simulink model "SystemComposerModel"  (R2022b)
settings: Solver=VariableStepAuto  StartTime=0.0  StopTime=10.0  RelTol=1e-3
(part 2 of 3)

== system SystemComposerModel/Crazyflie 2.0/Results ==
  Bus Element In1 : Inport  PortName=Tests
  ResultsAnalysis : Subsystem
      settings: PortSchema="{\"entries\":[{\"content\":{\"headerSize\":26,\"margin\":15,\"minimumSpacing\":25,\"sides\":[{\"content\":{\"connectorIds\":[\"In1\"]},\"type\":\"ConnectorPlacement.EquallySpacedRectSide\",\"uuid\":\"b8d7d09c-e9ae-43de-8d46-f99ec2351e24\"},{\"content\":{\"connectorIds\":[\"Out1\"],\"side\":\"RIGHT\"},\"type\":\"ConnectorPlacement.EquallySpacedRectSide\",\"uuid\":\"4693648e-b0a2-4db8-a983-4bee2f51d894\"},{\"content\":{\"connectorIds\":[],\"side\":\"TOP\"},\"type\":\"ConnectorPlacement.EquallySpacedRectSide\",\"uuid\":\"9f0e5fe3-4fa7-4597-a4df-94b2d5032736\"}]},\"type\":\"ConnectorPlacement.EquallySpacedConnector\",\"uuid\":\"297bf07a-4341-4423-8aed-0af6edbe7857\"}],\"packageUris\":[\"http://schema.mathworks.com/mf0/Connector/R2020b\"],\"version\":\"1.0\"}"
  Bus Element Out1 : Outport  PortName=CodeModifications
  wires:
  Bus Element In1/1 -> ResultsAnalysis/1(Tests)
  ResultsAnalysis/1(CodeModifications) -> Bus Element Out1/1

== system SystemComposerModel/Crazyflie 2.0/STEM ranging ==
  Bus Element Out1 : Outport  PortName=dist_front
  Bus Element Out2 : Outport  Port=2  PortName=dist_rear
  Bus Element Out3 : Outport  Port=3  PortName=dist_right
  Bus Element Out4 : Outport  Port=4  PortName=dist_left

== system SystemComposerModel/Crazyflie 2.0/State Estimator ==
  Bus Element In1 : Inport  PortName=Current state
  Bus Element In2 : Inport  Port=2  PortName=Actuation Signal
  Bus Element Out1 : Outport  PortName=Estimated State

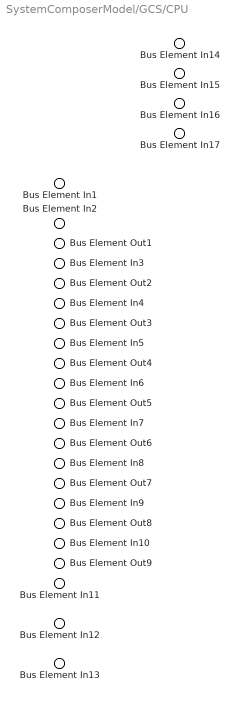
== system SystemComposerModel/GCS/CPU ==
  Bus Element In17 : Inport  PortName=CodeModifications
  Bus Element In14 : Inport  Port=2  PortName=F_x_in
  Bus Element In15 : Inport  Port=3  PortName=F_y_in
  Bus Element In16 : Inport  Port=4  PortName=F_z_in
  Bus Element In1 : Inport  Port=5  PortName=pos_x_in
  Bus Element In2 : Inport  Port=6  PortName=pos_y_in
  Bus Element In3 : Inport  Port=7  PortName=pos_z_in
  Bus Element In4 : Inport  Port=8  PortName=alpha_in
  Bus Element In5 : Inport  Port=9  PortName=beta_in
  Bus Element In6 : Inport  Port=10  PortName=gamma_in
  Bus Element In7 : Inport  Port=11  PortName=vel_x_in
  Bus Element In8 : Inport  Port=12  PortName=vel_y_in
  Bus Element In9 : Inport  Port=13  PortName=vel_z_in
  Bus Element In10 : Inport  Port=14  PortName=Obst_x1_in
  Bus Element In11 : Inport  Port=15  PortName=Obst_y1_in
  Bus Element In12 : Inport  Port=16  PortName=Obst_x2_in
  Bus Element In13 : Inport  Port=17  PortName=Obst_y2_in
  Bus Element Out1 : Outport  PortName=pos_x_out
  Bus Element Out2 : Outport  Port=2  PortName=pos_y_out
  Bus Element Out3 : Outport  Port=3  PortName=pos_z_out
  Bus Element Out4 : Outport  Port=4  PortName=alpha_out
  Bus Element Out5 : Outport  Port=5  PortName=beta_out
  Bus Element Out6 : Outport  Port=6  PortName=gamma_out
  Bus Element Out7 : Outport  Port=7  PortName=vel_x_out
  Bus Element Out8 : Outport  Port=8  PortName=vel_y_out
  Bus Element Out9 : Outport  Port=9  PortName=vel_z_out

== system SystemComposerModel/GCS/ClimConditions ==
  Bus Element In1 : Inport  PortName=Enviroment
  Wind : Subsystem
      settings: PortSchema="{\"entries\":[{\"content\":{\"headerSize\":26,\"margin\":15,\"minimumSpacing\":25,\"sides\":[{\"content\":{\"connectorIds\":[\"In1\"]},\"type\":\"ConnectorPlacement.EquallySpacedRectSide\",\"uuid\":\"b8d7d09c-e9ae-43de-8d46-f99ec2351e24\"},{\"content\":{\"connectorIds\":[\"Out1\",\"Out2\",\"Out3\"],\"side\":\"RIGHT\"},\"type\":\"ConnectorPlacement.EquallySpacedRectSide\",\"uuid\":\"4693648e-b0a2-4db8-a983-4bee2f51d894\"},{\"content\":{\"connectorIds\":[],\"side\":\"TOP\"},\"type\":\"ConnectorPlacement.EquallySpacedRectSide\",\"uuid\":\"9f0e5fe3-4fa7-4597-a4df-94b2d5032736\"}]},\"type\":\"ConnectorPlacement.EquallySpacedConnector\",\"uuid\":\"297bf07a-4341-4423-8aed-0af6edbe7857\"}],\"packageUris\":[\"http://schema.mathworks.com/mf0/Connector/R2020b\"],\"version\":\"1.0\"}"
  Bus Element Out1 : Outport  PortName=F_x_in
  Bus Element Out2 : Outport  Port=2  PortName=F_y_in
  Bus Element Out3 : Outport  Port=3  PortName=F_z_in
  wires:
  Bus Element In1/1 -> Wind/1(Enviroment)
  Wind/1(F_x_in) -> Bus Element Out1/1
  Wind/2(F_y_in) -> Bus Element Out2/1
  Wind/3(F_z_in) -> Bus Element Out3/1

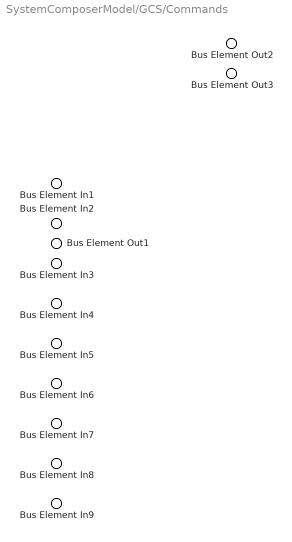
== system SystemComposerModel/GCS/Commands ==
  Bus Element In1 : Inport  PortName=pos_x_out
  Bus Element In2 : Inport  Port=2  PortName=pos_y_out
  Bus Element In3 : Inport  Port=3  PortName=pos_z_out
  Bus Element In4 : Inport  Port=4  PortName=alpha_out
  Bus Element In5 : Inport  Port=5  PortName=beta_out
  Bus Element In6 : Inport  Port=6  PortName=gamma_out
  Bus Element In7 : Inport  Port=7  PortName=vel_x_out
  Bus Element In8 : Inport  Port=8  PortName=vel_y_out
  Bus Element In9 : Inport  Port=9  PortName=vel_z_out
  Bus Element Out2 : Outport  PortName=Telemetry_USB
  Bus Element Out3 : Outport  Port=2  PortName=TelemetryFeedback
  Bus Element Out1 : Outport  Port=3  PortName=GCSCmds

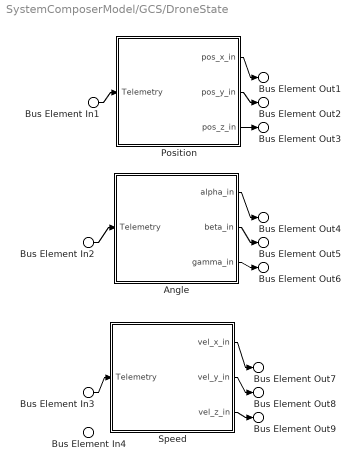
== system SystemComposerModel/GCS/DroneState ==
  Bus Element In1 : Inport  PortName=Telemetry
  Bus Element In2 : Inport  PortName=Telemetry
  Bus Element In3 : Inport  PortName=Telemetry
  Bus Element In4 : Inport  Port=2  PortName=TelemetryFeedback
  Angle : Subsystem
      settings: PortSchema="{\"entries\":[{\"content\":{\"headerSize\":26,\"margin\":15,\"minimumSpacing\":25,\"sides\":[{\"content\":{\"connectorIds\":[\"In1\"]},\"type\":\"ConnectorPlacement.EquallySpacedRectSide\",\"uuid\":\"b8d7d09c-e9ae-43de-8d46-f99ec2351e24\"},{\"content\":{\"connectorIds\":[\"Out1\",\"Out2\",\"Out3\"],\"side\":\"RIGHT\"},\"type\":\"ConnectorPlacement.EquallySpacedRectSide\",\"uuid\":\"4693648e-b0a2-4db8-a983-4bee2f51d894\"},{\"content\":{\"connectorIds\":[],\"side\":\"TOP\"},\"type\":\"ConnectorPlacement.EquallySpacedRectSide\",\"uuid\":\"9f0e5fe3-4fa7-4597-a4df-94b2d5032736\"}]},\"type\":\"ConnectorPlacement.EquallySpacedConnector\",\"uuid\":\"297bf07a-4341-4423-8aed-0af6edbe7857\"}],\"packageUris\":[\"http://schema.mathworks.com/mf0/Connector/R2020b\"],\"version\":\"1.0\"}"
  Position : Subsystem
      settings: PortSchema="{\"entries\":[{\"content\":{\"headerSize\":26,\"margin\":15,\"minimumSpacing\":25,\"sides\":[{\"content\":{\"connectorIds\":[\"In1\"]},\"type\":\"ConnectorPlacement.EquallySpacedRectSide\",\"uuid\":\"b8d7d09c-e9ae-43de-8d46-f99ec2351e24\"},{\"content\":{\"connectorIds\":[\"Out1\",\"Out2\",\"Out3\"],\"side\":\"RIGHT\"},\"type\":\"ConnectorPlacement.EquallySpacedRectSide\",\"uuid\":\"4693648e-b0a2-4db8-a983-4bee2f51d894\"},{\"content\":{\"connectorIds\":[],\"side\":\"TOP\"},\"type\":\"ConnectorPlacement.EquallySpacedRectSide\",\"uuid\":\"9f0e5fe3-4fa7-4597-a4df-94b2d5032736\"}]},\"type\":\"ConnectorPlacement.EquallySpacedConnector\",\"uuid\":\"297bf07a-4341-4423-8aed-0af6edbe7857\"}],\"packageUris\":[\"http://schema.mathworks.com/mf0/Connector/R2020b\"],\"version\":\"1.0\"}"
  Speed : Subsystem
      settings: PortSchema="{\"entries\":[{\"content\":{\"headerSize\":26,\"margin\":15,\"minimumSpacing\":25,\"sides\":[{\"content\":{\"connectorIds\":[\"In1\"]},\"type\":\"ConnectorPlacement.EquallySpacedRectSide\",\"uuid\":\"b8d7d09c-e9ae-43de-8d46-f99ec2351e24\"},{\"content\":{\"connectorIds\":[\"Out1\",\"Out2\",\"Out3\"],\"side\":\"RIGHT\"},\"type\":\"ConnectorPlacement.EquallySpacedRectSide\",\"uuid\":\"4693648e-b0a2-4db8-a983-4bee2f51d894\"},{\"content\":{\"connectorIds\":[],\"side\":\"TOP\"},\"type\":\"ConnectorPlacement.EquallySpacedRectSide\",\"uuid\":\"9f0e5fe3-4fa7-4597-a4df-94b2d5032736\"}]},\"type\":\"ConnectorPlacement.EquallySpacedConnector\",\"uuid\":\"297bf07a-4341-4423-8aed-0af6edbe7857\"}],\"packageUris\":[\"http://schema.mathworks.com/mf0/Connector/R2020b\"],\"version\":\"1.0\"}"
  Bus Element Out1 : Outport  PortName=pos_x_in
  Bus Element Out2 : Outport  Port=2  PortName=pos_y_in
  Bus Element Out3 : Outport  Port=3  PortName=pos_z_in
  Bus Element Out4 : Outport  Port=4  PortName=alpha_in
  Bus Element Out5 : Outport  Port=5  PortName=beta_in
  Bus Element Out6 : Outport  Port=6  PortName=gamma_in
  Bus Element Out7 : Outport  Port=7  PortName=vel_x_in
  Bus Element Out8 : Outport  Port=8  PortName=vel_y_in
  Bus Element Out9 : Outport  Port=9  PortName=vel_z_in
  wires:
  Bus Element In1/1 -> Position/1(Telemetry)
  Bus Element In2/1 -> Angle/1(Telemetry)
  Bus Element In3/1 -> Speed/1(Telemetry)
  Position/1(pos_x_in) -> Bus Element Out1/1
  Position/2(pos_y_in) -> Bus Element Out2/1
  Position/3(pos_z_in) -> Bus Element Out3/1
  Angle/1(alpha_in) -> Bus Element Out4/1
  Angle/2(beta_in) -> Bus Element Out5/1
  Angle/3(gamma_in) -> Bus Element Out6/1
  Speed/1(vel_x_in) -> Bus Element Out7/1
  Speed/2(vel_y_in) -> Bus Element Out8/1
  Speed/3(vel_z_in) -> Bus Element Out9/1

== system SystemComposerModel/GCS/References ==
  Bus Element In1 : Inport  PortName=FPVVideo
  ObstacleDetection : Subsystem
      settings: PortSchema="{\"entries\":[{\"content\":{\"headerSize\":26,\"margin\":15,\"minimumSpacing\":25,\"sides\":[{\"content\":{\"connectorIds\":[\"In1\"]},\"type\":\"ConnectorPlacement.EquallySpacedRectSide\",\"uuid\":\"b8d7d09c-e9ae-43de-8d46-f99ec2351e24\"},{\"content\":{\"connectorIds\":[\"Out1\",\"Out2\",\"Out3\",\"Out4\"],\"side\":\"RIGHT\"},\"type\":\"ConnectorPlacement.EquallySpacedRectSide\",\"uuid\":\"4693648e-b0a2-4db8-a983-4bee2f51d894\"},{\"content\":{\"connectorIds\":[],\"side\":\"TOP\"},\"type\":\"ConnectorPlacement.EquallySpacedRectSide\",\"uuid\":\"9f0e5fe3-4fa7-4597-a4df-94b2d5032736\"}]},\"type\":\"ConnectorPlacement.EquallySpacedConnector\",\"uuid\":\"297bf07a-4341-4423-8aed-0af6edbe7857\"}],\"packageUris\":[\"http://schema.mathworks.com/mf0/Connector/R2020b\"],\"version\":\"1.0\"}"
  Bus Element Out4 : Outport  PortName=Obst_x1_in
  Bus Element Out2 : Outport  Port=2  PortName=Obst_y1_in
  Bus Element Out3 : Outport  Port=3  PortName=Obst_x2_in
  Bus Element Out1 : Outport  Port=4  PortName=Obst_y2_in
  wires:
  Bus Element In1/1 -> ObstacleDetection/1(FPVVideo)
  ObstacleDetection/4(Obst_y2_in) -> Bus Element Out1/1
  ObstacleDetection/3(Obst_y1_in) -> Bus Element Out2/1
  ObstacleDetection/2(Obst_x2_in) -> Bus Element Out3/1
  ObstacleDetection/1(Obst_x1_in) -> Bus Element Out4/1

== system SystemComposerModel/GCS/Results ==
  Bus Element In1 : Inport  PortName=Tests
  ResultsAnalysis : Subsystem
      settings: PortSchema="{\"entries\":[{\"content\":{\"headerSize\":26,\"margin\":15,\"minimumSpacing\":25,\"sides\":[{\"content\":{\"connectorIds\":[\"In1\"]},\"type\":\"ConnectorPlacement.EquallySpacedRectSide\",\"uuid\":\"b8d7d09c-e9ae-43de-8d46-f99ec2351e24\"},{\"content\":{\"connectorIds\":[\"Out1\"],\"side\":\"RIGHT\"},\"type\":\"ConnectorPlacement.EquallySpacedRectSide\",\"uuid\":\"4693648e-b0a2-4db8-a983-4bee2f51d894\"},{\"content\":{\"connectorIds\":[],\"side\":\"TOP\"},\"type\":\"ConnectorPlacement.EquallySpacedRectSide\",\"uuid\":\"9f0e5fe3-4fa7-4597-a4df-94b2d5032736\"}]},\"type\":\"ConnectorPlacement.EquallySpacedConnector\",\"uuid\":\"297bf07a-4341-4423-8aed-0af6edbe7857\"}],\"packageUris\":[\"http://schema.mathworks.com/mf0/Connector/R2020b\"],\"version\":\"1.0\"}"
  Bus Element Out1 : Outport  PortName=CodeModifications
  wires:
  Bus Element In1/1 -> ResultsAnalysis/1(Tests)
  ResultsAnalysis/1(CodeModifications) -> Bus Element Out1/1

== system SystemComposerModel/Competition/Materials/Advertising ==
  Bus Element Out1 : Outport  PortName=Marketing

== system SystemComposerModel/Competition/Materials/Chronometer ==

== system SystemComposerModel/Competition/Materials/Horn ==
  Bus Element Out1 : Outport  PortName=Start

== system SystemComposerModel/Competition/Materials/Insulating tapes ==
  Bus Element Out1 : Outport  PortName=Lines

== system SystemComposerModel/Competition/Materials/Obstacles ==
  Doors : Subsystem  Description=They must be overcome by passing through the middle. The doors will be 1x1 meter square and elevated with the lower base half a meter off the ground.
      settings: PortSchema="{\"entries\":[{\"content\":{\"headerSize\":26,\"margin\":15,\"minimumSpacing\":25,\"sides\":[{\"content\":{\"connectorIds\":[]},\"type\":\"ConnectorPlacement.EquallySpacedRectSide\",\"uuid\":\"9053b2a7-4775-4bcf-9fc6-a069826350a9\"},{\"content\":{\"connectorIds\":[],\"side\":\"RIGHT\"},\"type\":\"ConnectorPlacement.EquallySpacedRectSide\",\"uuid\":\"b0969818-a4d3-4cbe-99b6-1949e99be80f\"},{\"content\":{\"connectorIds\":[],\"side\":\"TOP\"},\"type\":\"ConnectorPlacement.EquallySpacedRectSide\",\"uuid\":\"6c494ee9-6eb7-4ac7-893f-bc2d7701a0da\"}]},\"type\":\"ConnectorPlacement.EquallySpacedConnector\",\"uuid\":\"7a7eacf3-349d-4601-bac9-f57d73c6d0e2\"}],\"packageUris\":[\"http://schema.mathworks.com/mf0/Connector/R2020b\"],\"version\":\"1.0\"}"
  Split Rectangle : Subsystem  Description=They can be red or blue. If they are red, you pass over them and if they are blue, you pass under them. The whole surface of the obstacle will be the same color and each rectangle will be 2x1m.
      settings: PortSchema="{\"entries\":[{\"content\":{\"headerSize\":26,\"margin\":15,\"minimumSpacing\":25,\"sides\":[{\"content\":{\"connectorIds\":[]},\"type\":\"ConnectorPlacement.EquallySpacedRectSide\",\"uuid\":\"9053b2a7-4775-4bcf-9fc6-a069826350a9\"},{\"content\":{\"connectorIds\":[\"Out1\"],\"side\":\"RIGHT\"},\"type\":\"ConnectorPlacement.EquallySpacedRectSide\",\"uuid\":\"b0969818-a4d3-4cbe-99b6-1949e99be80f\"},{\"content\":{\"connectorIds\":[],\"side\":\"TOP\"},\"type\":\"ConnectorPlacement.EquallySpacedRectSide\",\"uuid\":\"6c494ee9-6eb7-4ac7-893f-bc2d7701a0da\"}]},\"type\":\"ConnectorPlacement.EquallySpacedConnector\",\"uuid\":\"7a7eacf3-349d-4601-bac9-f57d73c6d0e2\"}],\"packageUris\":[\"http://schema.mathworks.com/mf0/Connector/R2020b\"],\"version\":\"1.0\"}"
  Sticks : Subsystem  Description=They can be red or blue. If they are red they are passed on the left and if they are blue on the right. The stick will be 1.5 meters long and 4 cm wide. For a correct overcoming of the obstacle, the drone must not move more than 0.5 meters away from the sides and cannot exceed the height of the stick.
      settings: PortSchema="{\"entries\":[{\"content\":{\"headerSize\":26,\"margin\":15,\"minimumSpacing\":25,\"sides\":[{\"content\":{\"connectorIds\":[]},\"type\":\"ConnectorPlacement.EquallySpacedRectSide\",\"uuid\":\"9053b2a7-4775-4bcf-9fc6-a069826350a9\"},{\"content\":{\"connectorIds\":[],\"side\":\"RIGHT\"},\"type\":\"ConnectorPlacement.EquallySpacedRectSide\",\"uuid\":\"b0969818-a4d3-4cbe-99b6-1949e99be80f\"},{\"content\":{\"connectorIds\":[],\"side\":\"TOP\"},\"type\":\"ConnectorPlacement.EquallySpacedRectSide\",\"uuid\":\"6c494ee9-6eb7-4ac7-893f-bc2d7701a0da\"}]},\"type\":\"ConnectorPlacement.EquallySpacedConnector\",\"uuid\":\"7a7eacf3-349d-4601-bac9-f57d73c6d0e2\"}],\"packageUris\":[\"http://schema.mathworks.com/mf0/Connector/R2020b\"],\"version\":\"1.0\"}"
  Bus Element Out1 : Outport  PortName=obs
  wires:
  Split Rectangle/1(OutBus) -> Bus Element Out1/1

== system SystemComposerModel/Competition/Materials/Projector ==
  Bus Element Out1 : Outport  PortName=Proyection

== system SystemComposerModel/Competition/Organization/Before the competition ==
  Marketing : Subsystem  Description=Tasks related to the marketing of the event. Must be started at most 2 weeks before the event.
      settings: PortSchema="{\"entries\":[{\"content\":{\"headerSize\":26,\"margin\":15,\"minimumSpacing\":25,\"sides\":[{\"content\":{\"connectorIds\":[]},\"type\":\"ConnectorPlacement.EquallySpacedRectSide\",\"uuid\":\"d34c32ef-3d27-469b-8a35-abebe5333993\"},{\"content\":{\"connectorIds\":[],\"side\":\"RIGHT\"},\"type\":\"ConnectorPlacement.EquallySpacedRectSide\",\"uuid\":\"0a2917af-f234-4cdf-997c-680a118988b7\"},{\"content\":{\"connectorIds\":[],\"side\":\"TOP\"},\"type\":\"ConnectorPlacement.EquallySpacedRectSide\",\"uuid\":\"dcac7d54-9fff-4582-ba14-08bcbac36cd8\"}]},\"type\":\"ConnectorPlacement.EquallySpacedConnector\",\"uuid\":\"84591ee6-ffcc-49ff-97f7-997353b331d9\"}],\"packageUris\":[\"http://schema.mathworks.com/mf0/Connector/R2020b\"],\"version\":\"1.0\"}"
  Space reservation : Subsystem  Description=Must be done 2 month before the start of the event.
      settings: PortSchema="{\"entries\":[{\"content\":{\"headerSize\":26,\"margin\":15,\"minimumSpacing\":25,\"sides\":[{\"content\":{\"connectorIds\":[]},\"type\":\"ConnectorPlacement.EquallySpacedRectSide\",\"uuid\":\"d34c32ef-3d27-469b-8a35-abebe5333993\"},{\"content\":{\"connectorIds\":[],\"side\":\"RIGHT\"},\"type\":\"ConnectorPlacement.EquallySpacedRectSide\",\"uuid\":\"0a2917af-f234-4cdf-997c-680a118988b7\"},{\"content\":{\"connectorIds\":[],\"side\":\"TOP\"},\"type\":\"ConnectorPlacement.EquallySpacedRectSide\",\"uuid\":\"dcac7d54-9fff-4582-ba14-08bcbac36cd8\"}]},\"type\":\"ConnectorPlacement.EquallySpacedConnector\",\"uuid\":\"84591ee6-ffcc-49ff-97f7-997353b331d9\"}],\"packageUris\":[\"http://schema.mathworks.com/mf0/Connector/R2020b\"],\"version\":\"1.0\"}"

== system SystemComposerModel/Competition/Organization/During the competition ==
  Date : Subsystem  Description=To be defined. It will be at the end of the course.
      settings: PortSchema="{\"entries\":[{\"content\":{\"headerSize\":26,\"margin\":15,\"minimumSpacing\":25,\"sides\":[{\"content\":{\"connectorIds\":[]},\"type\":\"ConnectorPlacement.EquallySpacedRectSide\",\"uuid\":\"d34c32ef-3d27-469b-8a35-abebe5333993\"},{\"content\":{\"connectorIds\":[],\"side\":\"RIGHT\"},\"type\":\"ConnectorPlacement.EquallySpacedRectSide\",\"uuid\":\"0a2917af-f234-4cdf-997c-680a118988b7\"},{\"content\":{\"connectorIds\":[],\"side\":\"TOP\"},\"type\":\"ConnectorPlacement.EquallySpacedRectSide\",\"uuid\":\"dcac7d54-9fff-4582-ba14-08bcbac36cd8\"}]},\"type\":\"ConnectorPlacement.EquallySpacedConnector\",\"uuid\":\"84591ee6-ffcc-49ff-97f7-997353b331d9\"}],\"packageUris\":[\"http://schema.mathworks.com/mf0/Connector/R2020b\"],\"version\":\"1.0\"}"
  Place : Subsystem  Description=Place of the event. It will be the sports centre of ETSII.
      settings: PortSchema="{\"entries\":[{\"content\":{\"headerSize\":26,\"margin\":15,\"minimumSpacing\":25,\"sides\":[{\"content\":{\"connectorIds\":[]},\"type\":\"ConnectorPlacement.EquallySpacedRectSide\",\"uuid\":\"d34c32ef-3d27-469b-8a35-abebe5333993\"},{\"content\":{\"connectorIds\":[],\"side\":\"RIGHT\"},\"type\":\"ConnectorPlacement.EquallySpacedRectSide\",\"uuid\":\"0a2917af-f234-4cdf-997c-680a118988b7\"},{\"content\":{\"connectorIds\":[],\"side\":\"TOP\"},\"type\":\"ConnectorPlacement.EquallySpacedRectSide\",\"uuid\":\"dcac7d54-9fff-4582-ba14-08bcbac36cd8\"}]},\"type\":\"ConnectorPlacement.EquallySpacedConnector\",\"uuid\":\"84591ee6-ffcc-49ff-97f7-997353b331d9\"}],\"packageUris\":[\"http://schema.mathworks.com/mf0/Connector/R2020b\"],\"version\":\"1.0\"}"
  Schedule : Subsystem  Description=The schedule for the different activities of the event. To be defined.
      settings: PortSchema="{\"entries\":[{\"content\":{\"headerSize\":26,\"margin\":15,\"minimumSpacing\":25,\"sides\":[{\"content\":{\"connectorIds\":[]},\"type\":\"ConnectorPlacement.EquallySpacedRectSide\",\"uuid\":\"d34c32ef-3d27-469b-8a35-abebe5333993\"},{\"content\":{\"connectorIds\":[],\"side\":\"RIGHT\"},\"type\":\"ConnectorPlacement.EquallySpacedRectSide\",\"uuid\":\"0a2917af-f234-4cdf-997c-680a118988b7\"},{\"content\":{\"connectorIds\":[],\"side\":\"TOP\"},\"type\":\"ConnectorPlacement.EquallySpacedRectSide\",\"uuid\":\"dcac7d54-9fff-4582-ba14-08bcbac36cd8\"}]},\"type\":\"ConnectorPlacement.EquallySpacedConnector\",\"uuid\":\"84591ee6-ffcc-49ff-97f7-997353b331d9\"}],\"packageUris\":[\"http://schema.mathworks.com/mf0/Connector/R2020b\"],\"version\":\"1.0\"}"

== system SystemComposerModel/Competition/People/Audience ==

== system SystemComposerModel/Competition/People/Observers ==

== system SystemComposerModel/Competition/People/Participants ==

== system SystemComposerModel/Competition/Trials/Prueba 1: Speed ==
  Bus Element In1 : Inport  PortName=Start
  Rules : Subsystem  Description=|
      | The two drones will compete simultaneously, at a distance of at least 5 meters from each other and from the enclosure boundaries.
      | No AI deck or camera is required in this test. 
      | Take-off when the start signal is given, which will consist of a horn sound.
      | Collision between drones means expulsion from the test of the drone that has deviated from the straight line (can be both).
      | The drones must be able to brake so as not to collide with the end of the pavilion. The contestants will calculate the time of power-on of the drone taking into account its maximum speed and the length of the pavilion.
      | Landing after braking.
      | The drone will be disqualified from the test if it takes off before the horn.
      | A time keeper from each team will be stationed at the end of the straight with a stopwatch to mark the finish time. If there is a difference of more than 0.3s between stopwatches the race will be repeated (to avoid cheating).
      settings: PortSchema="{\"entries\":[{\"content\":{\"headerSize\":26,\"margin\":15,\"minimumSpacing\":25,\"sides\":[{\"content\":{\"connectorIds\":[]},\"type\":\"ConnectorPlacement.EquallySpacedRectSide\",\"uuid\":\"9053b2a7-4775-4bcf-9fc6-a069826350a9\"},{\"content\":{\"connectorIds\":[],\"side\":\"RIGHT\"},\"type\":\"ConnectorPlacement.EquallySpacedRectSide\",\"uuid\":\"b0969818-a4d3-4cbe-99b6-1949e99be80f\"},{\"content\":{\"connectorIds\":[],\"side\":\"TOP\"},\"type\":\"ConnectorPlacement.EquallySpacedRectSide\",\"uuid\":\"6c494ee9-6eb7-4ac7-893f-bc2d7701a0da\"}]},\"type\":\"ConnectorPlacement.EquallySpacedConnector\",\"uuid\":\"7a7eacf3-349d-4601-bac9-f57d73c6d0e2\"}],\"packageUris\":[\"http://schema.mathworks.com/mf0/Connector/R2020b\"],\"version\":\"1.0\"}"
  Scoring : Subsystem  Description=|
      | The correct take-off/landing will be analyzed.
      | In this test what determines the score is the time that separates the landing from the take-off, having traveled the length of the pavilion between both maneuvers.
      | The first drone to land after crossing the finish line is considered the winner.
      | A score of 20 points will be awarded to the winning drone and 10 to the losing drone, regardless of the difference that may exist in the times of one and the other. In case of a tie, 15 points will be given to each.
      settings: PortSchema="{\"entries\":[{\"content\":{\"headerSize\":26,\"margin\":15,\"minimumSpacing\":25,\"sides\":[{\"content\":{\"connectorIds\":[]},\"type\":\"ConnectorPlacement.EquallySpacedRectSide\",\"uuid\":\"9053b2a7-4775-4bcf-9fc6-a069826350a9\"},{\"content\":{\"connectorIds\":[],\"side\":\"RIGHT\"},\"type\":\"ConnectorPlacement.EquallySpacedRectSide\",\"uuid\":\"b0969818-a4d3-4cbe-99b6-1949e99be80f\"},{\"content\":{\"connectorIds\":[],\"side\":\"TOP\"},\"type\":\"ConnectorPlacement.EquallySpacedRectSide\",\"uuid\":\"6c494ee9-6eb7-4ac7-893f-bc2d7701a0da\"}]},\"type\":\"ConnectorPlacement.EquallySpacedConnector\",\"uuid\":\"7a7eacf3-349d-4601-bac9-f57d73c6d0e2\"}],\"packageUris\":[\"http://schema.mathworks.com/mf0/Connector/R2020b\"],\"version\":\"1.0\"}"

== system SystemComposerModel/Competition/Trials/Prueba 2: Diana ==
  Bus Element In1 : Inport  PortName=Proyection
  Rules : Subsystem  Description=|
      | Drone takes off when it sees green light on the projector, the screen will turn green for 5 seconds, and the drone will be waiting for the circles.
      | Drone lands when it sees red light on the screen, the screen will turn red for 5 seconds.
      | During 1 minute, one by one black filled circles of 10 cm diameter will be projected consecutively on a wall in an area of 3x2 meters. Each circle will be visible between 4 and 8 seconds, and its position will not be known beforehand but will be the same for both teams.
      | The projector will be 2 meters away from the wall and on the floor, at an angle that makes the projection possible and leaving the drone a maneuvering area such that it does not get in front of the projector.
      | The drone will be disqualified from the event if it covers the projector.
      | Two observers, one from each team, will count the hits. The laser must stay at least an appreciable time inside the circle to count as a hit, it is not enough to pass over it as it may be chance and not the result of the drone's computation.
      settings: PortSchema="{\"entries\":[{\"content\":{\"headerSize\":26,\"margin\":15,\"minimumSpacing\":25,\"sides\":[{\"content\":{\"connectorIds\":[]},\"type\":\"ConnectorPlacement.EquallySpacedRectSide\",\"uuid\":\"9053b2a7-4775-4bcf-9fc6-a069826350a9\"},{\"content\":{\"connectorIds\":[],\"side\":\"RIGHT\"},\"type\":\"ConnectorPlacement.EquallySpacedRectSide\",\"uuid\":\"b0969818-a4d3-4cbe-99b6-1949e99be80f\"},{\"content\":{\"connectorIds\":[],\"side\":\"TOP\"},\"type\":\"ConnectorPlacement.EquallySpacedRectSide\",\"uuid\":\"6c494ee9-6eb7-4ac7-893f-bc2d7701a0da\"}]},\"type\":\"ConnectorPlacement.EquallySpacedConnector\",\"uuid\":\"7a7eacf3-349d-4601-bac9-f57d73c6d0e2\"}],\"packageUris\":[\"http://schema.mathworks.com/mf0/Connector/R2020b\"],\"version\":\"1.0\"}"
  Scoring : Subsystem  Description=|
      | Highest number of hits while aiming at the target.
      | Disqualification in case of obstructing the projection of the targets.
      | The maximum score of the test is 20 points.
      | In this test all the circles will have the same score, so that 20/x points will be added (x being the number of total circles that will appear) each time the laser is placed on a circle at least the stipulated time. 
      | Even if a drone gets the score for a certain circle, the other drone will also be able to get the score for the same circle even if it has put its laser on it later.
      settings: PortSchema="{\"entries\":[{\"content\":{\"headerSize\":26,\"margin\":15,\"minimumSpacing\":25,\"sides\":[{\"content\":{\"connectorIds\":[]},\"type\":\"ConnectorPlacement.EquallySpacedRectSide\",\"uuid\":\"9053b2a7-4775-4bcf-9fc6-a069826350a9\"},{\"content\":{\"connectorIds\":[],\"side\":\"RIGHT\"},\"type\":\"ConnectorPlacement.EquallySpacedRectSide\",\"uuid\":\"b0969818-a4d3-4cbe-99b6-1949e99be80f\"},{\"content\":{\"connectorIds\":[],\"side\":\"TOP\"},\"type\":\"ConnectorPlacement.EquallySpacedRectSide\",\"uuid\":\"6c494ee9-6eb7-4ac7-893f-bc2d7701a0da\"}]},\"type\":\"ConnectorPlacement.EquallySpacedConnector\",\"uuid\":\"7a7eacf3-349d-4601-bac9-f57d73c6d0e2\"}],\"packageUris\":[\"http://schema.mathworks.com/mf0/Connector/R2020b\"],\"version\":\"1.0\"}"

== system SystemComposerModel/Competition/Trials/Prueba 3: Line following ==
  Bus Element In2 : Inport  PortName=Líneas
  Bus Element In1 : Inport  Port=2  PortName=Start
  Rules : Subsystem  Description=|
      | The drone takes off when the start signal is given, which will consist of a horn sound.
      | The drone must follow a continuous black line 38mm wide from start to finish. 
      | The drone must pass through checkpoints (to be defined when the circuit is created) to avoid cheating shortcuts.
      | The circuit will not be known by the teams in advance, it will be random.
      | There will be two types of possible bifurcations:
      | Thinner black line, representing a distraction to avoid, 10mm wide.
      | Red line 20mm wide, which represents the optimal route, thus giving a higher score.
      | The lines shall be sufficiently far apart so as not to confuse the camera.
      | Lines may not cross each other.
      | Landing when a blue tape mark is detected.
      settings: PortSchema="{\"entries\":[{\"content\":{\"headerSize\":26,\"margin\":15,\"minimumSpacing\":25,\"sides\":[{\"content\":{\"connectorIds\":[]},\"type\":\"ConnectorPlacement.EquallySpacedRectSide\",\"uuid\":\"9053b2a7-4775-4bcf-9fc6-a069826350a9\"},{\"content\":{\"connectorIds\":[],\"side\":\"RIGHT\"},\"type\":\"ConnectorPlacement.EquallySpacedRectSide\",\"uuid\":\"b0969818-a4d3-4cbe-99b6-1949e99be80f\"},{\"content\":{\"connectorIds\":[],\"side\":\"TOP\"},\"type\":\"ConnectorPlacement.EquallySpacedRectSide\",\"uuid\":\"6c494ee9-6eb7-4ac7-893f-bc2d7701a0da\"}]},\"type\":\"ConnectorPlacement.EquallySpacedConnector\",\"uuid\":\"7a7eacf3-349d-4601-bac9-f57d73c6d0e2\"}],\"packageUris\":[\"http://schema.mathworks.com/mf0/Connector/R2020b\"],\"version\":\"1.0\"}"
  Scoring : Subsystem  Description=|
      | In this test, drones are awarded points for following a line. When the drone leaves the line it will be given the score of the last control point; from that moment on it is not possible to continue scoring even if the drone recovers the trajectory of the line.
      | To run the complete circuit through the thickest lines possible will result in obtaining the maximum possible score in the test, which will be 18 points.
      | The thickness of the line indicates the score that gives a given section to the next control point. To obtain the score, the area of the lines traversed (thickness * length) is calculated, multiplied by 18 and divided by the area of the lines of the highest scoring path.
      | If you land correctly, you will get 2 extra points, so you can get up to 20 points in this test.
      settings: PortSchema="{\"entries\":[{\"content\":{\"headerSize\":26,\"margin\":15,\"minimumSpacing\":25,\"sides\":[{\"content\":{\"connectorIds\":[]},\"type\":\"ConnectorPlacement.EquallySpacedRectSide\",\"uuid\":\"9053b2a7-4775-4bcf-9fc6-a069826350a9\"},{\"content\":{\"connectorIds\":[],\"side\":\"RIGHT\"},\"type\":\"ConnectorPlacement.EquallySpacedRectSide\",\"uuid\":\"b0969818-a4d3-4cbe-99b6-1949e99be80f\"},{\"content\":{\"connectorIds\":[],\"side\":\"TOP\"},\"type\":\"ConnectorPlacement.EquallySpacedRectSide\",\"uuid\":\"6c494ee9-6eb7-4ac7-893f-bc2d7701a0da\"}]},\"type\":\"ConnectorPlacement.EquallySpacedConnector\",\"uuid\":\"7a7eacf3-349d-4601-bac9-f57d73c6d0e2\"}],\"packageUris\":[\"http://schema.mathworks.com/mf0/Connector/R2020b\"],\"version\":\"1.0\"}"

== system SystemComposerModel/Competition/Trials/Prueba 4: Predefined Obstacles ==
  Bus Element In2 : Inport  PortName=Start
  Bus Element In1 : Inport  Port=2  PortName=Obstacles
  Rules : Subsystem  Description=|
      | Take-off when the departure signal is given, which will consist of a horn sound.
      | Landing when the bidi code of the last obstacle is detected.
      | Provided there is no obstacle present, the drone should be kept at a height of approximately 1m.
      | If an obstacle is omitted it will be considered erroneous.
      | The route must be completed in less than 4 minutes.
      settings: PortSchema="{\"entries\":[{\"content\":{\"headerSize\":26,\"margin\":15,\"minimumSpacing\":25,\"sides\":[{\"content\":{\"connectorIds\":[]},\"type\":\"ConnectorPlacement.EquallySpacedRectSide\",\"uuid\":\"9053b2a7-4775-4bcf-9fc6-a069826350a9\"},{\"content\":{\"connectorIds\":[],\"side\":\"RIGHT\"},\"type\":\"ConnectorPlacement.EquallySpacedRectSide\",\"uuid\":\"b0969818-a4d3-4cbe-99b6-1949e99be80f\"},{\"content\":{\"connectorIds\":[],\"side\":\"TOP\"},\"type\":\"ConnectorPlacement.EquallySpacedRectSide\",\"uuid\":\"6c494ee9-6eb7-4ac7-893f-bc2d7701a0da\"}]},\"type\":\"ConnectorPlacement.EquallySpacedConnector\",\"uuid\":\"7a7eacf3-349d-4601-bac9-f57d73c6d0e2\"}],\"packageUris\":[\"http://schema.mathworks.com/mf0/Connector/R2020b\"],\"version\":\"1.0\"}"
  Scoring : Subsystem  Description=|
      | Test with obstacles (predefined and random): the score at the start of the race is zero points. 
      | Each obstacle passed adds one point. 
      | If the time between two obstacles of one team is at least 0.25 seconds shorter than the time between the same obstacles of the other team, the team with the shorter time will score an additional point (to avoid very close results, where the reaction time of the observers is very important). 
      | To measure the times, two observers will be designated (one of them will be an observer). Two observers (one from each team) will be designated for each obstacle. Their function will be to time the moment when the drone crosses the obstacle. At the start of the race, all observers will start a stopwatch on their mobile devices and stop it when the drone passes the obstacle. If the difference between the times of the two observers is less than 0.2 seconds, the average of the two times will be taken. If this is not the case, this time will not be taken into account for both teams, but the time between two non-consecutive obstacles (with the invalidated one in between) will be taken into account.
      settings: PortSchema="{\"entries\":[{\"content\":{\"headerSize\":26,\"margin\":15,\"minimumSpacing\":25,\"sides\":[{\"content\":{\"connectorIds\":[]},\"type\":\"ConnectorPlacement.EquallySpacedRectSide\",\"uuid\":\"9053b2a7-4775-4bcf-9fc6-a069826350a9\"},{\"content\":{\"connectorIds\":[],\"side\":\"RIGHT\"},\"type\":\"ConnectorPlacement.EquallySpacedRectSide\",\"uuid\":\"b0969818-a4d3-4cbe-99b6-1949e99be80f\"},{\"content\":{\"connectorIds\":[],\"side\":\"TOP\"},\"type\":\"ConnectorPlacement.EquallySpacedRectSide\",\"uuid\":\"6c494ee9-6eb7-4ac7-893f-bc2d7701a0da\"}]},\"type\":\"ConnectorPlacement.EquallySpacedConnector\",\"uuid\":\"7a7eacf3-349d-4601-bac9-f57d73c6d0e2\"}],\"packageUris\":[\"http://schema.mathworks.com/mf0/Connector/R2020b\"],\"version\":\"1.0\"}"
  Trial Obstacles : Subsystem
      settings: PortSchema="{\"entries\":[{\"content\":{\"headerSize\":26,\"margin\":15,\"minimumSpacing\":25,\"sides\":[{\"content\":{\"connectorIds\":[\"In1\"]},\"type\":\"ConnectorPlacement.EquallySpacedRectSide\",\"uuid\":\"9053b2a7-4775-4bcf-9fc6-a069826350a9\"},{\"content\":{\"connectorIds\":[],\"side\":\"RIGHT\"},\"type\":\"ConnectorPlacement.EquallySpacedRectSide\",\"uuid\":\"b0969818-a4d3-4cbe-99b6-1949e99be80f\"},{\"content\":{\"connectorIds\":[],\"side\":\"TOP\"},\"type\":\"ConnectorPlacement.EquallySpacedRectSide\",\"uuid\":\"6c494ee9-6eb7-4ac7-893f-bc2d7701a0da\"}]},\"type\":\"ConnectorPlacement.EquallySpacedConnector\",\"uuid\":\"7a7eacf3-349d-4601-bac9-f57d73c6d0e2\"}],\"packageUris\":[\"http://schema.mathworks.com/mf0/Connector/R2020b\"],\"version\":\"1.0\"}"
  wires:
  Bus Element In1/1 -> Trial Obstacles/1(Obstacles)

== system SystemComposerModel/Competition/Trials/Prueba 5: Random obstacles ==
  Bus Element In2 : Inport  PortName=Start
  Bus Element In1 : Inport  Port=2  PortName=Obstacles
  Rules : Subsystem  Description=|
      | The obstacles will be random.
      | Take-off when the start signal is given, which will consist of a horn sound.
      | Landing when the bidi code of the last obstacle is detected.
      | Test with obstacles (predefined and random): the score at the start of the race is zero points. 
      | Each obstacle passed adds one point. 
      | If the time between two obstacles of one team is at least 0.25 seconds less than the time between the same obstacles of the other team, the team with the shorter time will score an additional point (to avoid very close results, where the reaction time of the observers is very important). 
      | To measure the times, two observers will be designated (one of them will be an observer). Two observers (one from each team) will be designated for each obstacle. Their function will be to time the moment when the drone crosses the obstacle. At the start of the race, all observers will start a stopwatch on their mobile devices and stop it when the drone passes the obstacle. If the difference between the times of the two observers is less than 0.2 seconds, the average of the two times will be taken. If this is not the case, this time will not be taken into account for both teams, but the time between two non-consecutive obstacles (with the invalidated one in between) will be taken into account.
      settings: PortSchema="{\"entries\":[{\"content\":{\"headerSize\":26,\"margin\":15,\"minimumSpacing\":25,\"sides\":[{\"content\":{\"connectorIds\":[]},\"type\":\"ConnectorPlacement.EquallySpacedRectSide\",\"uuid\":\"9053b2a7-4775-4bcf-9fc6-a069826350a9\"},{\"content\":{\"connectorIds\":[],\"side\":\"RIGHT\"},\"type\":\"ConnectorPlacement.EquallySpacedRectSide\",\"uuid\":\"b0969818-a4d3-4cbe-99b6-1949e99be80f\"},{\"content\":{\"connectorIds\":[],\"side\":\"TOP\"},\"type\":\"ConnectorPlacement.EquallySpacedRectSide\",\"uuid\":\"6c494ee9-6eb7-4ac7-893f-bc2d7701a0da\"}]},\"type\":\"ConnectorPlacement.EquallySpacedConnector\",\"uuid\":\"7a7eacf3-349d-4601-bac9-f57d73c6d0e2\"}],\"packageUris\":[\"http://schema.mathworks.com/mf0/Connector/R2020b\"],\"version\":\"1.0\"}"
  Scoring : Subsystem  Description=|
      | Test with obstacles (predefined and random): the score at the start of the race is zero points. 
      | Each obstacle passed adds one point. 
      | If the time between two obstacles of one team is at least 0.25 seconds shorter than the time between the same obstacles of the other team, the team with the shorter time will score an additional point (to avoid very close results, where the reaction time of the observers is very important). 
      | To measure the times, two observers will be designated (one of them will be an observer). Two observers (one from each team) will be designated for each obstacle. Their function will be to time the moment when the drone crosses the obstacle. At the start of the race, all observers will start a stopwatch on their mobile devices and stop it when the drone passes the obstacle. If the difference between the times of the two observers is less than 0.2 seconds, the average of the two times will be taken. If this is not the case, this time will not be taken into account for both teams, but the time between two non-consecutive obstacles (with the invalidated one in between) will be taken into account.
      settings: PortSchema="{\"entries\":[{\"content\":{\"headerSize\":26,\"margin\":15,\"minimumSpacing\":25,\"sides\":[{\"content\":{\"connectorIds\":[]},\"type\":\"ConnectorPlacement.EquallySpacedRectSide\",\"uuid\":\"9053b2a7-4775-4bcf-9fc6-a069826350a9\"},{\"content\":{\"connectorIds\":[],\"side\":\"RIGHT\"},\"type\":\"ConnectorPlacement.EquallySpacedRectSide\",\"uuid\":\"b0969818-a4d3-4cbe-99b6-1949e99be80f\"},{\"content\":{\"connectorIds\":[],\"side\":\"TOP\"},\"type\":\"ConnectorPlacement.EquallySpacedRectSide\",\"uuid\":\"6c494ee9-6eb7-4ac7-893f-bc2d7701a0da\"}]},\"type\":\"ConnectorPlacement.EquallySpacedConnector\",\"uuid\":\"7a7eacf3-349d-4601-bac9-f57d73c6d0e2\"}],\"packageUris\":[\"http://schema.mathworks.com/mf0/Connector/R2020b\"],\"version\":\"1.0\"}"
  Trial Obstacles1 : Subsystem
      settings: PortSchema="{\"entries\":[{\"content\":{\"headerSize\":26,\"margin\":15,\"minimumSpacing\":25,\"sides\":[{\"content\":{\"connectorIds\":[\"In1\"]},\"type\":\"ConnectorPlacement.EquallySpacedRectSide\",\"uuid\":\"9053b2a7-4775-4bcf-9fc6-a069826350a9\"},{\"content\":{\"connectorIds\":[],\"side\":\"RIGHT\"},\"type\":\"ConnectorPlacement.EquallySpacedRectSide\",\"uuid\":\"b0969818-a4d3-4cbe-99b6-1949e99be80f\"},{\"content\":{\"connectorIds\":[],\"side\":\"TOP\"},\"type\":\"ConnectorPlacement.EquallySpacedRectSide\",\"uuid\":\"6c494ee9-6eb7-4ac7-893f-bc2d7701a0da\"}]},\"type\":\"ConnectorPlacement.EquallySpacedConnector\",\"uuid\":\"7a7eacf3-349d-4601-bac9-f57d73c6d0e2\"}],\"packageUris\":[\"http://schema.mathworks.com/mf0/Connector/R2020b\"],\"version\":\"1.0\"}"

== system SystemComposerModel/Competition/Trials/Prueba 6: Freestyle ==
  Bus Element In1 : Inport  PortName=Start
  Rules : Subsystem  Description=Both teams will perform it separately.
      settings: PortSchema="{\"entries\":[{\"content\":{\"headerSize\":26,\"margin\":15,\"minimumSpacing\":25,\"sides\":[{\"content\":{\"connectorIds\":[]},\"type\":\"ConnectorPlacement.EquallySpacedRectSide\",\"uuid\":\"9053b2a7-4775-4bcf-9fc6-a069826350a9\"},{\"content\":{\"connectorIds\":[],\"side\":\"RIGHT\"},\"type\":\"ConnectorPlacement.EquallySpacedRectSide\",\"uuid\":\"b0969818-a4d3-4cbe-99b6-1949e99be80f\"},{\"content\":{\"connectorIds\":[],\"side\":\"TOP\"},\"type\":\"ConnectorPlacement.EquallySpacedRectSide\",\"uuid\":\"6c494ee9-6eb7-4ac7-893f-bc2d7701a0da\"}]},\"type\":\"ConnectorPlacement.EquallySpacedConnector\",\"uuid\":\"7a7eacf3-349d-4601-bac9-f57d73c6d0e2\"}],\"packageUris\":[\"http://schema.mathworks.com/mf0/Connector/R2020b\"],\"version\":\"1.0\"}"

== system SystemComposerModel/Crazyflie 2.0/ClimConditions/Wind ==
  Bus Element In1 : Inport  PortName=Enviroment
  Bus Element Out1 : Outport  PortName=F_x_in
  Bus Element Out2 : Outport  Port=2  PortName=F_y_in
  Bus Element Out3 : Outport  Port=3  PortName=F_z_in

== system SystemComposerModel/Crazyflie 2.0/Results/ResultsAnalysis ==
  Bus Element In1 : Inport  PortName=Tests
  Bus Element Out1 : Outport  PortName=CodeModifications

== system SystemComposerModel/GCS/ClimConditions/Wind ==
  Bus Element In1 : Inport  PortName=Enviroment
  Bus Element Out1 : Outport  PortName=F_x_in
  Bus Element Out2 : Outport  Port=2  PortName=F_y_in
  Bus Element Out3 : Outport  Port=3  PortName=F_z_in

== system SystemComposerModel/GCS/DroneState/Angle ==
  Bus Element In1 : Inport  PortName=Telemetry
  Bus Element Out1 : Outport  PortName=alpha_in
  Bus Element Out2 : Outport  Port=2  PortName=beta_in
  Bus Element Out3 : Outport  Port=3  PortName=gamma_in

== system SystemComposerModel/GCS/DroneState/Position ==
  Bus Element In1 : Inport  PortName=Telemetry
  Bus Element Out1 : Outport  PortName=pos_x_in
  Bus Element Out2 : Outport  Port=2  PortName=pos_y_in
  Bus Element Out3 : Outport  Port=3  PortName=pos_z_in

== system SystemComposerModel/GCS/DroneState/Speed ==
  Bus Element In1 : Inport  PortName=Telemetry
  Bus Element Out1 : Outport  PortName=vel_x_in
  Bus Element Out2 : Outport  Port=2  PortName=vel_y_in
  Bus Element Out3 : Outport  Port=3  PortName=vel_z_in

== system SystemComposerModel/GCS/References/ObstacleDetection ==
  Bus Element In1 : Inport  PortName=FPVVideo
  Bus Element Out1 : Outport  PortName=Obst_x1_in
  Bus Element Out2 : Outport  Port=2  PortName=Obst_x2_in
  Bus Element Out3 : Outport  Port=3  PortName=Obst_y1_in
  Bus Element Out4 : Outport  Port=4  PortName=Obst_y2_in

== system SystemComposerModel/GCS/Results/ResultsAnalysis ==
  Bus Element In1 : Inport  PortName=Tests
  Bus Element Out1 : Outport  PortName=CodeModifications

== system SystemComposerModel/Competition/Materials/Obstacles/Doors ==

== system SystemComposerModel/Competition/Materials/Obstacles/Split Rectangle ==
  Bus Element Out1 : Outport  PortName=OutBus

== system SystemComposerModel/Competition/Materials/Obstacles/Sticks ==

== system SystemComposerModel/Competition/Organization/Before the competition/Marketing ==

== system SystemComposerModel/Competition/Organization/Before the competition/Space reservation ==

== system SystemComposerModel/Competition/Organization/During the competition/Date ==

== system SystemComposerModel/Competition/Organization/During the competition/Place ==

== system SystemComposerModel/Competition/Organization/During the competition/Schedule ==

== system SystemComposerModel/Competition/Trials/Prueba 1: Speed/Rules ==

== system SystemComposerModel/Competition/Trials/Prueba 1: Speed/Scoring ==

== system SystemComposerModel/Competition/Trials/Prueba 2: Diana/Rules ==

== system SystemComposerModel/Competition/Trials/Prueba 2: Diana/Scoring ==

== system SystemComposerModel/Competition/Trials/Prueba 3: Line following/Rules ==

== system SystemComposerModel/Competition/Trials/Prueba 3: Line following/Scoring ==

== system SystemComposerModel/Competition/Trials/Prueba 4: Predefined Obstacles/Rules ==

== system SystemComposerModel/Competition/Trials/Prueba 4: Predefined Obstacles/Scoring ==

== system SystemComposerModel/Competition/Trials/Prueba 4: Predefined Obstacles/Trial Obstacles ==
  Bus Element In1 : Inport  PortName=Obstacles
  Doors : Subsystem  Description=They must be overcome by passing through the middle. The doors will be 1x1 meter square and elevated with the lower base half a meter off the ground.
      settings: PortSchema="{\"entries\":[{\"content\":{\"headerSize\":26,\"margin\":15,\"minimumSpacing\":25,\"sides\":[{\"content\":{\"connectorIds\":[]},\"type\":\"ConnectorPlacement.EquallySpacedRectSide\",\"uuid\":\"9053b2a7-4775-4bcf-9fc6-a069826350a9\"},{\"content\":{\"connectorIds\":[],\"side\":\"RIGHT\"},\"type\":\"ConnectorPlacement.EquallySpacedRectSide\",\"uuid\":\"b0969818-a4d3-4cbe-99b6-1949e99be80f\"},{\"content\":{\"connectorIds\":[],\"side\":\"TOP\"},\"type\":\"ConnectorPlacement.EquallySpacedRectSide\",\"uuid\":\"6c494ee9-6eb7-4ac7-893f-bc2d7701a0da\"}]},\"type\":\"ConnectorPlacement.EquallySpacedConnector\",\"uuid\":\"7a7eacf3-349d-4601-bac9-f57d73c6d0e2\"}],\"packageUris\":[\"http://schema.mathworks.com/mf0/Connector/R2020b\"],\"version\":\"1.0\"}"
  Split rectangle : Subsystem  Description=They can be red or blue. If they are red, you pass over them and if they are blue, you pass under them. The whole surface of the obstacle will be the same color and each rectangle will be 2x1m.
      settings: PortSchema="{\"entries\":[{\"content\":{\"headerSize\":26,\"margin\":15,\"minimumSpacing\":25,\"sides\":[{\"content\":{\"connectorIds\":[]},\"type\":\"ConnectorPlacement.EquallySpacedRectSide\",\"uuid\":\"9053b2a7-4775-4bcf-9fc6-a069826350a9\"},{\"content\":{\"connectorIds\":[],\"side\":\"RIGHT\"},\"type\":\"ConnectorPlacement.EquallySpacedRectSide\",\"uuid\":\"b0969818-a4d3-4cbe-99b6-1949e99be80f\"},{\"content\":{\"connectorIds\":[],\"side\":\"TOP\"},\"type\":\"ConnectorPlacement.EquallySpacedRectSide\",\"uuid\":\"6c494ee9-6eb7-4ac7-893f-bc2d7701a0da\"}]},\"type\":\"ConnectorPlacement.EquallySpacedConnector\",\"uuid\":\"7a7eacf3-349d-4601-bac9-f57d73c6d0e2\"}],\"packageUris\":[\"http://schema.mathworks.com/mf0/Connector/R2020b\"],\"version\":\"1.0\"}"
  Sticks : Subsystem  Description=They can be red or blue. If they are red they are passed on the left and if they are blue on the right. The stick will be 1.5 meters long and 4 cm wide. For a correct overcoming of the obstacle, the drone must not move more than 0.5 meters away from the sides and cannot exceed the height of the stick.
      settings: PortSchema="{\"entries\":[{\"content\":{\"headerSize\":26,\"margin\":15,\"minimumSpacing\":25,\"sides\":[{\"content\":{\"connectorIds\":[]},\"type\":\"ConnectorPlacement.EquallySpacedRectSide\",\"uuid\":\"9053b2a7-4775-4bcf-9fc6-a069826350a9\"},{\"content\":{\"connectorIds\":[],\"side\":\"RIGHT\"},\"type\":\"ConnectorPlacement.EquallySpacedRectSide\",\"uuid\":\"b0969818-a4d3-4cbe-99b6-1949e99be80f\"},{\"content\":{\"connectorIds\":[],\"side\":\"TOP\"},\"type\":\"ConnectorPlacement.EquallySpacedRectSide\",\"uuid\":\"6c494ee9-6eb7-4ac7-893f-bc2d7701a0da\"}]},\"type\":\"ConnectorPlacement.EquallySpacedConnector\",\"uuid\":\"7a7eacf3-349d-4601-bac9-f57d73c6d0e2\"}],\"packageUris\":[\"http://schema.mathworks.com/mf0/Connector/R2020b\"],\"version\":\"1.0\"}"

== system SystemComposerModel/Competition/Trials/Prueba 5: Random obstacles/Rules ==

== system SystemComposerModel/Competition/Trials/Prueba 5: Random obstacles/Scoring ==
